simulink model "BTC"  (R2024b)
settings: Solver=FixedStepAuto  StartTime=0.0  StopTime=inf  FixedStep=btck_stepSize  RelTol=1e-3  EnableMultiTasking=on
values from neighbouring files (symbols this model uses):
  btcc_ambient_temp_highth = 45    [BTC_init.m]
  btcc_ambient_temp_lowth = -30    [BTC_init.m]
  btcc_cell_temp_diffth = 5    [BTC_init.m]
  btcc_full_soc = 95    [BTC_init.m]
  btcc_Ki = 0.5    [BTC_init.m]
  btcc_Kp = 2    [BTC_init.m]
  btcc_max_temp_highth = 40    [BTC_init.m]
  btcc_max_temp_lowth = 35    [BTC_init.m]
  btcc_min_temp_highth = 25    [BTC_init.m]
  btcc_min_temp_lowth = 20    [BTC_init.m]
  btcc_number_in_series = 40    [BTC_init.m]
  btcc_pack_in_parallel = 1    [BTC_init.m]
  btck_stepSize = 0.1    [BTC_init.m]
undefined symbols (not defined in the file or in its folder): DiscIntNeverNeededParam
settings Model: Creator=favv5g  LastModifiedBy=voillat
settings ConfigSet: Description=OpenECU configuration set for code generation under RTW-EC.
settings SolverCC: AlgebraicLoopSolver=TrustRegion  PositivePriorityOrder=on
settings DataIOCC: LimitDataPoints=on  SaveFormat=Array  SignalLoggingSaveFormat=ModelDataLogs
settings OptimizationCC: DefaultParameterBehavior=Inlined  InlineInvariantSignals=on  ExpressionDepthLimit=2147483647  StateBitsets=on  DataBitsets=on  ZeroExternalMemoryAtStartup=off  ZeroInternalMemoryAtStartup=off  NoFixptDivByZeroProtection=on  EfficientFloat2IntCast=on  LifeSpan=1  EfficientTunableParamExpr=on
settings DebuggingCC: SaveWithParameterizedLinksMsg=none  SignalResolutionControl=TryResolveAllWithWarning  MultiTaskDSMMsg=warning  MultiTaskCondExecSysMsg=none  SingleTaskRateTransMsg=error  CheckMatrixSingularityMsg=warning  VectorMatrixConversionMsg=warning  SignalLabelMismatchMsg=warning  UnconnectedInputMsg=warning  UnconnectedOutputMsg=warning  UnconnectedLineMsg=warning  AllowSymbolicDim=off  StateNameClashWarn=warning  SFUnexpectedBacktrackingDiag=warning  SFNoUnconditionalDefaultTransitionDiag=warning  SFExecutionAtInitializationDiag=none  ArithmeticOperatorsInVariantConditions=warning
settings HardwareCC: ProdBitPerPointer=32  ProdBitPerSizeT=32  ProdBitPerPtrDiffT=32  ProdLargestAtomicInteger=Long  ProdLargestAtomicFloat=Double  ProdEndianess=BigEndian  ProdWordSize=32  ProdHWDeviceType=Freescale->32-bit PowerPC  TargetIntDivRoundTo=Zero  TargetEndianess=BigEndian  TargetHWDeviceType=Freescale->32-bit PowerPC  ProdEqTarget=off
settings ModelReferenceCC: EnableRefExpFcnMdlSchedulingChecks=on  PropagateSignalLabelsOutOfModel=off
settings SFSimCC: SimUseLocalCustomCode=off  MATLABDynamicMemAlloc=off  CustomCodeUndefinedFunction=UseInterfaceOnly
settings RTWCC: Description=OpenECU Platform Target (ERT, optimised floating-point code)  SystemTargetFile=openecu_ert.tlc  MakeCommand=make_rtw optimized_floating_point=1  TemplateMakefile=openecu_ert_r2015b_64.tmf  RetainRTWFile=on  RTWUseLocalCustomCode=off  IncludeHyperlinkInReport=on  GPUComputeCapability=3.5
settings CodeAppCC: ForceParamTrailComments=on  IgnoreCustomStorageClasses=off  SimulinkDataObjDesc=on  CustomSymbolStrType=$N$R$M  InsertBlockDesc=on  StateflowObjectComments=on  InternalIdentifier=Classic
settings STFCustomTargetCC: TargetLibSuffix=.a  GenerateSampleERTMain=on  IncludeMdlTerminateFcn=off  CombineOutputUpdateFcns=on  IncludeFileDelimiter=UseQuote  ERTCustomFileBanners=on  SupportContinuousTime=off  RemoveResetFunc=on  MATLABClassNameForMDSCustomization=Simulink.SoftwareTarget.ERTCustomization  SystemTargetFile=openecu_ert.tlc
settings ERTTargetCC: MultiwordLength=2048  GenerateSampleERTMain=on  ParMdlRefBuildCompliant=off  CompOptLevelCompliant=off  ConcurrentExecutionCompliant=off  IncludeMdlTerminateFcn=off  IncludeFileDelimiter=UseQuote  SupportNonInlinedSFcns=on  ModelStepFunctionPrototypeControlCompliant=off  CPPClassGenCompliant=off  UseToolchainInfoCompliant=off  ExtModeMexFile=noextcomm  ERTSrcFileBannerTemplate=oe_code_c_template.cgt  ERTHdrFileBannerTemplate=oe_code_h_template.cgt  ERTDataSrcFileTemplate=oe_data_c_template.cgt  ERTDataHdrFileTemplate=oe_data_h_template.cgt  ERTCustomFileTemplate=example_file_process.tlc  GlobalDataDefinition=InSeparateSourceFile  GlobalDataReference=InSeparateHeaderFile  ConvertIfToSwitch=off  SuppressUnreachableDefaultCases=off  EnableUserReplacementTypes=on  DynamicArrayContainerType=coder::array
settings ConfigComp: CovMetricSettings=dw  CovSaveCumulativeToWorkspaceVar=on  CovSaveSingleToWorkspaceVar=on  CovExternalEMLEnable=off

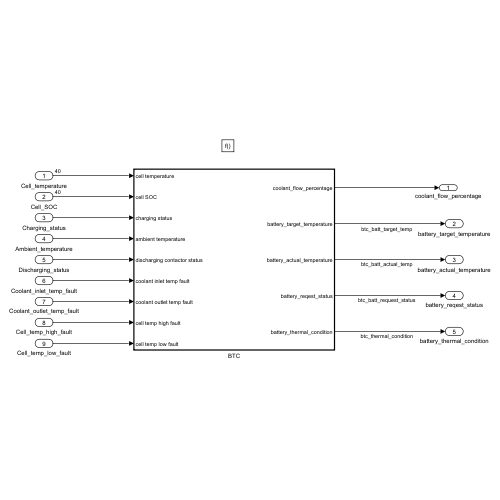
[thumbnail: Simulink's stored preview of the top-level diagram]
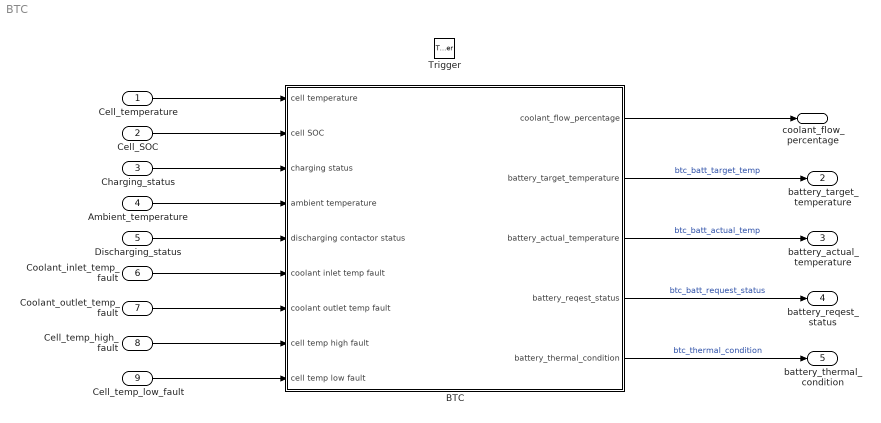
== system BTC ==
  Cell_temperature : Inport  PortDimensions=40
  Cell_SOC : Inport  Port=2  PortDimensions=40
  Charging_status : Inport  Port=3
  Ambient_temperature : Inport  Port=4
  Discharging_status : Inport  Port=5
  Coolant_inlet_temp_fault : Inport  Port=6
  Coolant_outlet_temp_fault : Inport  Port=7
  Cell_temp_high_fault : Inport  Port=8
  Cell_temp_low_fault : Inport  Port=9
  Trigger : TriggerPort  TriggerType=function-call  VariantControl=(inherit)  PortDimensions=1
  BTC : Subsystem  TreatAsAtomicUnit=on
  coolant_flow_percentage : Outport  VectorParamsAs1DForOutWhenUnconnected=off
  battery_target_temperature : Outport  Port=2  VectorParamsAs1DForOutWhenUnconnected=off
  battery_actual_temperature : Outport  Port=3  VectorParamsAs1DForOutWhenUnconnected=off
  battery_reqest_status : Outport  Port=4  VectorParamsAs1DForOutWhenUnconnected=off
  battery_thermal_condition : Outport  Port=5  VectorParamsAs1DForOutWhenUnconnected=off
  wires:
  BTC/1(coolant_flow_percentage) -> coolant_flow_percentage/1
  Cell_temperature/1 -> BTC/1(cell temperature)
  Cell_SOC/1 -> BTC/2(cell SOC)
  Charging_status/1 -> BTC/3(charging status)
  Ambient_temperature/1 -> BTC/4(ambient temperature)
  Discharging_status/1 -> BTC/5(discharging contactor status)
  Coolant_inlet_temp_fault/1 -> BTC/6(coolant inlet temp fault)
  Coolant_outlet_temp_fault/1 -> BTC/7(coolant outlet temp fault)
  Cell_temp_high_fault/1 -> BTC/8(cell temp high fault)
  Cell_temp_low_fault/1 -> BTC/9(cell temp low fault)
  BTC/2(battery_target_temperature) -> battery_target_temperature/1  "btc_batt_target_temp"
  BTC/3(battery_actual_temperature) -> battery_actual_temperature/1  "btc_batt_actual_temp"
  BTC/4(battery_reqest_status) -> battery_reqest_status/1  "btc_batt_request_status"
  BTC/5(battery_thermal_condition) -> battery_thermal_condition/1  "btc_thermal_condition"

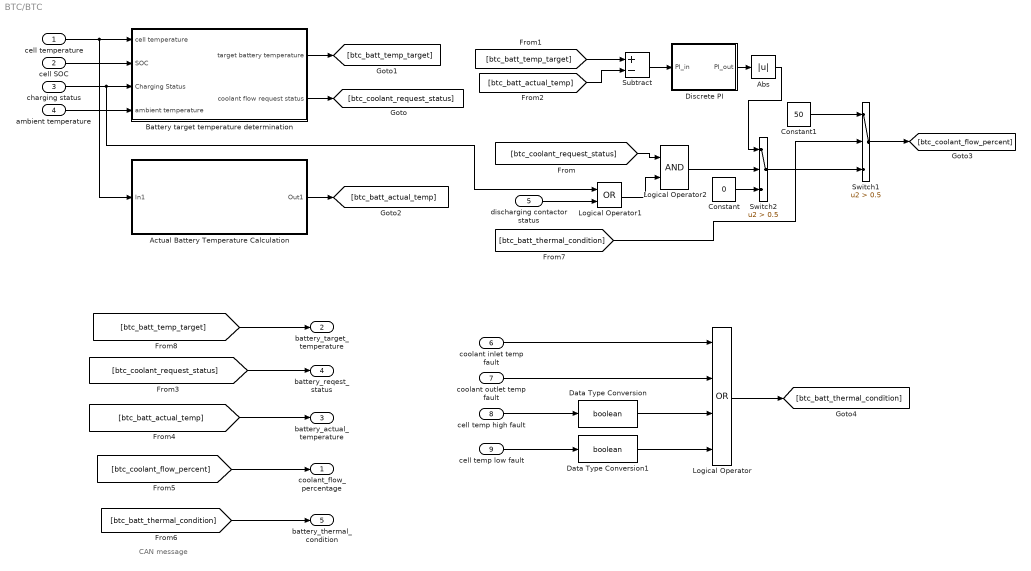
== system BTC/BTC ==
  note: CAN message
  cell temperature : Inport
  cell SOC : Inport  Port=2
  charging status : Inport  Port=3
  ambient temperature : Inport  Port=4
  discharging contactor status : Inport  Port=5
  coolant inlet temp fault : Inport  Port=6
  coolant outlet temp fault : Inport  Port=7
  cell temp high fault : Inport  Port=8  OutDataTypeStr=uint8
  cell temp low fault : Inport  Port=9  OutDataTypeStr=uint8
  Abs : Abs  SaturateOnIntegerOverflow=off
  Actual Battery Temperature Calculation : Subsystem
  Battery target temperature determination : Subsystem
  Constant : Constant  Value=0
  Constant1 : Constant  Value=50
  Data Type Conversion : DataTypeConversion  OutDataTypeStr=boolean  SaturateOnIntegerOverflow=off  RndMeth=Floor
  Data Type Conversion1 : DataTypeConversion  OutDataTypeStr=boolean  SaturateOnIntegerOverflow=off  RndMeth=Floor
  Discrete PI : Subsystem
  Logical Operator : Logic  Operator=OR  Inputs=4  AllPortsSameDT=off  OutDataTypeStr=boolean
  Logical Operator1 : Logic  Operator=OR  AllPortsSameDT=off  OutDataTypeStr=boolean
  Logical Operator2 : Logic  AllPortsSameDT=off  OutDataTypeStr=boolean
  Subtract : Sum  Inputs=+-
  Switch1 : Switch  Criteria=u2 > Threshold  Threshold=0.5  SaturateOnIntegerOverflow=off  InputSameDT=off
  Switch2 : Switch  Criteria=u2 > Threshold  Threshold=0.5  SaturateOnIntegerOverflow=off  InputSameDT=off
  coolant_flow_percentage : Outport  VectorParamsAs1DForOutWhenUnconnected=off
  battery_target_temperature : Outport  Port=2  VectorParamsAs1DForOutWhenUnconnected=off
  battery_actual_temperature : Outport  Port=3  VectorParamsAs1DForOutWhenUnconnected=off
  battery_reqest_status : Outport  Port=4  VectorParamsAs1DForOutWhenUnconnected=off
  battery_thermal_condition : Outport  Port=5  VectorParamsAs1DForOutWhenUnconnected=off
  wires:
  cell temperature/1 -> Actual Battery Temperature Calculation/1(In1), Battery target temperature determination/1(cell temperature)
  Constant/1 -> Switch2/3
  Battery target temperature determination/2(coolant flow request status) -> [btc_coolant_request_status]
  Battery target temperature determination/1(target battery temperature) -> [btc_batt_temp_target]
  Actual Battery Temperature Calculation/1(Out1) -> [btc_batt_actual_temp]
  cell SOC/1 -> Battery target temperature determination/2(SOC)
  charging status/1 -> Logical Operator1/1, Battery target temperature determination/3(Charging Status)
  ambient temperature/1 -> Battery target temperature determination/4(ambient temperature)
  [btc_batt_temp_target] -> Subtract/1
  [btc_batt_actual_temp] -> Subtract/2
  [btc_batt_actual_temp] -> battery_actual_temperature/1
  [btc_coolant_flow_percent] -> coolant_flow_percentage/1
  coolant inlet temp fault/1 -> Logical Operator/1
  coolant outlet temp fault/1 -> Logical Operator/2
  cell temp high fault/1 -> Data Type Conversion/1
  cell temp low fault/1 -> Data Type Conversion1/1
  discharging contactor status/1 -> Logical Operator1/2
  [btc_coolant_request_status] -> Logical Operator2/1
  Logical Operator1/1 -> Logical Operator2/2
  Logical Operator2/1 -> Switch2/2
  Logical Operator/1 -> [btc_batt_thermal_condition]
  [btc_batt_thermal_condition] -> battery_thermal_condition/1
  [btc_batt_thermal_condition] -> Switch1/2
  Switch1/1 -> [btc_coolant_flow_percent]
  [btc_batt_temp_target] -> battery_target_temperature/1
  [btc_coolant_request_status] -> battery_reqest_status/1
  Switch2/1 -> Switch1/3
  Constant1/1 -> Switch1/1
  Abs/1 -> Switch2/1
  Data Type Conversion/1 -> Logical Operator/3
  Data Type Conversion1/1 -> Logical Operator/4
  Subtract/1 -> Discrete PI/1(PI_in)
  Discrete PI/1(PI_out) -> Abs/1

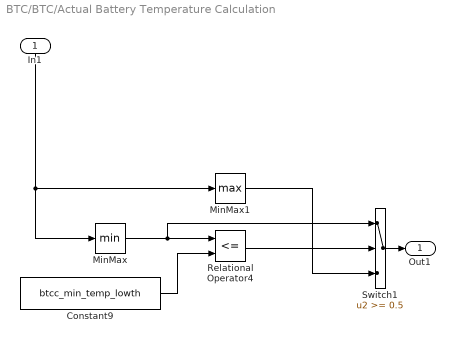
== system BTC/BTC/Actual Battery Temperature Calculation ==
  In1 : Inport
  Constant9 : Constant  Value=btcc_min_temp_lowth
  MinMax : MinMax
  MinMax1 : MinMax  Function=max
  Relational Operator4 : RelationalOperator  Operator=<=  OutDataTypeStr=boolean  InputSameDT=off
  Switch1 : Switch  Threshold=0.5  SaturateOnIntegerOverflow=off  InputSameDT=off
  Out1 : Outport  VectorParamsAs1DForOutWhenUnconnected=off
  wires:
  In1/1 -> MinMax/1, MinMax1/1
  MinMax/1 -> Switch1/1, Relational Operator4/1
  Constant9/1 -> Relational Operator4/2
  Switch1/1 -> Out1/1
  MinMax1/1 -> Switch1/3
  Relational Operator4/1 -> Switch1/2

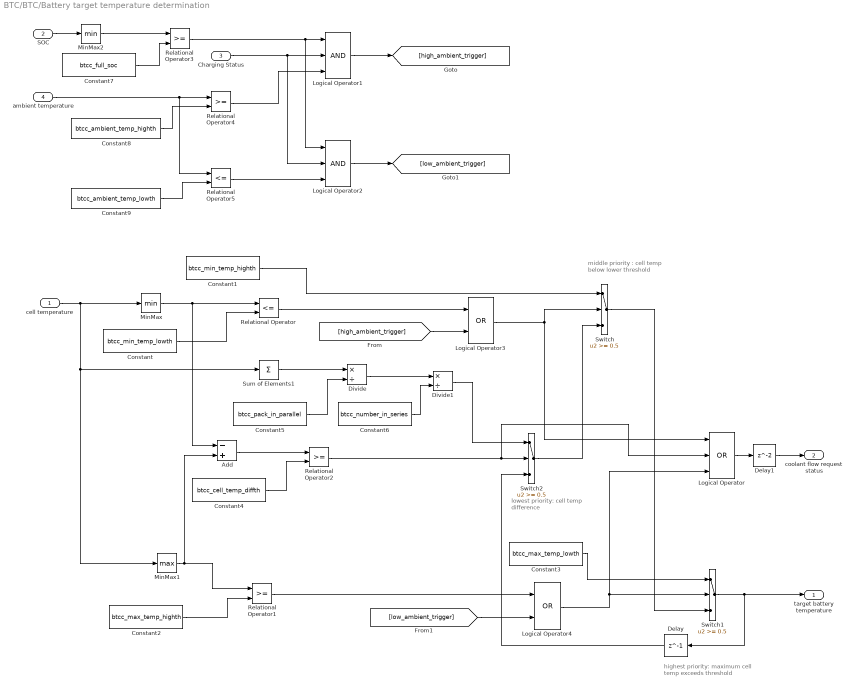
== system BTC/BTC/Battery target temperature determination ==
  note: middle priority : cell temp
      | below lower threshold
  note: highest priority: maximum cell
      | temp exceeds threshold
  note: lowest priority: cell
      | temp difference
  cell temperature : Inport
  SOC : Inport  Port=2
  Charging Status : Inport  Port=3
  ambient temperature : Inport  Port=4
  Add : Sum  Inputs=-+
  Constant : Constant  Value=btcc_min_temp_lowth
  Constant1 : Constant  Value=btcc_min_temp_highth
  Constant2 : Constant  Value=btcc_max_temp_highth
  Constant3 : Constant  Value=btcc_max_temp_lowth
  Constant4 : Constant  Value=btcc_cell_temp_diffth
  Constant5 : Constant  Value=btcc_pack_in_parallel
  Constant6 : Constant  Value=btcc_number_in_series
  Constant7 : Constant  Value=btcc_full_soc
  Constant8 : Constant  Value=btcc_ambient_temp_highth
  Constant9 : Constant  Value=btcc_ambient_temp_lowth
  Delay : Delay  DelayLength=1  InitialCondition=26
  Delay1 : Delay
  Divide : Product  Inputs=*/
  Divide1 : Product  Inputs=*/
  Logical Operator : Logic  Operator=OR  Inputs=3  AllPortsSameDT=off  OutDataTypeStr=boolean
  Logical Operator1 : Logic  Inputs=3  AllPortsSameDT=off  OutDataTypeStr=boolean
  Logical Operator2 : Logic  Inputs=3  AllPortsSameDT=off  OutDataTypeStr=boolean
  Logical Operator3 : Logic  Operator=OR  AllPortsSameDT=off  OutDataTypeStr=boolean
  Logical Operator4 : Logic  Operator=OR  AllPortsSameDT=off  OutDataTypeStr=boolean
  MinMax : MinMax
  MinMax1 : MinMax  Function=max
  MinMax2 : MinMax
  Relational Operator : RelationalOperator  Operator=<=  OutDataTypeStr=boolean  InputSameDT=off
  Relational Operator{1..4} (4 alike) : RelationalOperator  OutDataTypeStr=boolean  InputSameDT=off
  Relational Operator5 : RelationalOperator  Operator=<=  OutDataTypeStr=boolean  InputSameDT=off
  Sum of Elements1 : Sum  Inputs=+
  Switch : Switch  Threshold=0.5  SaturateOnIntegerOverflow=off  InputSameDT=off
  Switch1 : Switch  Threshold=0.5  SaturateOnIntegerOverflow=off  InputSameDT=off
  Switch2 : Switch  Threshold=0.5  SaturateOnIntegerOverflow=off  InputSameDT=off
  target battery temperature : Outport  VectorParamsAs1DForOutWhenUnconnected=off
  coolant flow request status : Outport  Port=2  VectorParamsAs1DForOutWhenUnconnected=off
  wires:
  cell temperature/1 -> MinMax/1, Sum of Elements1/1, MinMax1/1
  Constant/1 -> Relational Operator/2
  Constant2/1 -> Relational Operator1/2
  Constant3/1 -> Switch1/1
  Constant1/1 -> Switch/1
  MinMax1/1 -> Add/2, Relational Operator1/1
  MinMax/1 -> Add/1, Relational Operator/1
  Switch2/1 -> Switch/3
  Switch1/1 -> Delay/1, target battery temperature/1
  Switch/1 -> Switch1/3
  Constant4/1 -> Relational Operator2/2
  Add/1 -> Relational Operator2/1
  Sum of Elements1/1 -> Divide/1
  Constant5/1 -> Divide/2
  Divide/1 -> Divide1/1
  Constant6/1 -> Divide1/2
  Divide1/1 -> Switch2/1
  Relational Operator2/1 -> Switch2/2, Logical Operator/2
  Delay/1 -> Switch2/3
  SOC/1 -> MinMax2/1
  Constant7/1 -> Relational Operator3/2
  Charging Status/1 -> Logical Operator2/2, Logical Operator1/2
  Constant8/1 -> Relational Operator4/2
  Relational Operator4/1 -> Logical Operator1/3
  Logical Operator1/1 -> [high_ambient_trigger]
  Constant9/1 -> Relational Operator5/2
  Relational Operator5/1 -> Logical Operator2/3
  Relational Operator3/1 -> Logical Operator2/1, Logical Operator1/1
  Logical Operator2/1 -> [low_ambient_trigger]
  [high_ambient_trigger] -> Logical Operator3/2
  Logical Operator3/1 -> Logical Operator/1, Switch/2
  Relational Operator/1 -> Logical Operator3/1
  [low_ambient_trigger] -> Logical Operator4/2
  Relational Operator1/1 -> Logical Operator4/1
  Logical Operator4/1 -> Switch1/2, Logical Operator/3
  MinMax2/1 -> Relational Operator3/1
  ambient temperature/1 -> Relational Operator5/1, Relational Operator4/1
  Logical Operator/1 -> Delay1/1
  Delay1/1 -> coolant flow request status/1

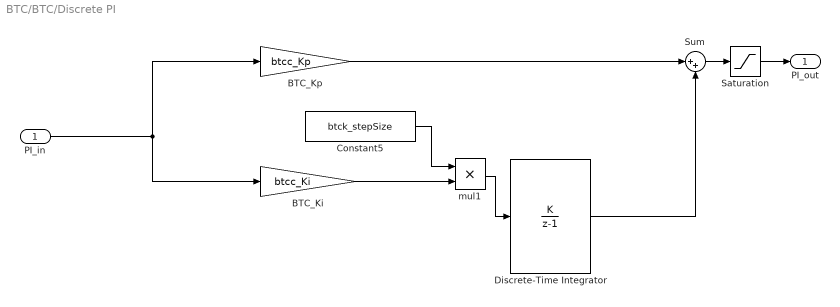
== system BTC/BTC/Discrete PI ==
  PI_in : Inport
  BTC_Ki : Gain  Gain=btcc_Ki
  BTC_Kp : Gain  Gain=btcc_Kp
  Constant5 : Constant  Value=btck_stepSize  SampleTime=-1
  Discrete-Time Integrator : DiscreteIntegrator  IntegratorMethod=Accumulation: Forward Euler  SampleTime=-1  UpperSaturationLimit=100  LowerSaturationLimit=-100  ICPrevOutput=DiscIntNeverNeededParam  ICPrevScaledInput=DiscIntNeverNeededParam
  Saturation : Saturate  UpperLimit=100  LowerLimit=-100
  Sum : Sum  Inputs=|++
  mul1 : Product  Inputs=**
  PI_out : Outport  VectorParamsAs1DForOutWhenUnconnected=off
  wires:
  PI_in/1 -> BTC_Ki/1, BTC_Kp/1
  Constant5/1 -> mul1/1
  BTC_Ki/1 -> mul1/2
  mul1/1 -> Discrete-Time Integrator/1
  BTC_Kp/1 -> Sum/1
  Discrete-Time Integrator/1 -> Sum/2
  Sum/1 -> Saturation/1
  Saturation/1 -> PI_out/1
